simulink model "NORTest"  (R2016a)
settings: Solver=VariableStepAuto  StartTime=0.0  StopTime=1  RelTol=1e-3
libraries: SimscapeMacros x5, elec_lib x2, fl_lib x1, ProjectBlocks x1, nesl_utility x1
settings Model: Creator=Peter  LastModifiedBy=Peter

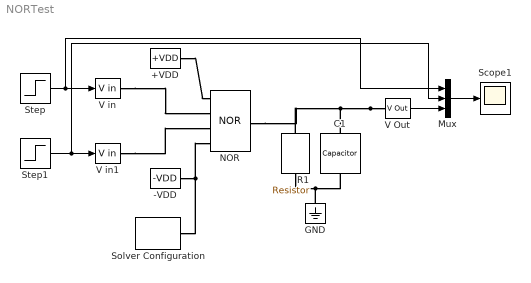
== system NORTest ==
  +VDD : SimscapeMacros/+VDD
  -VDD : SimscapeMacros/-VDD
  C1 : elec_lib/Passive Devices/Capacitor  enable_table=0  c=1e-6 F  Cvec=[ 1e-5 1e-6 ] F  Vvec=[ 0 10 ] V  CV_table_symmetry=1  C_tol=5  enable_C_tol=0  tol_distribution=1  nSigma=4  r=1e-6 Ohm  g=0 1/Ohm  initV=0 V  enable_operating_limits=0  operating_limit_action=1  max_working_voltage_range=[ -25 25 ] V  power_rating=1 W  enable_faults=0  fault_action=1  Cscale_faulted=100  R_faulted=0.001 Ohm  G_faulted=0 1/Ohm  tau_fault=0.001 s  enable_temporal_fault=0  t_fault=1 s  enable_behavioral_fault=0  max_permissible_voltage_range=[ -100 100 ] V  t_fail_on_voltage=1 s
  GND : fl_lib/Electrical/Electrical Elements/Electrical Reference
  Mux : Mux  Inputs=3
  NOR : ProjectBlocks/NOR
  R1 : elec_lib/Passive Devices/Resistor  R=10e3 Ohm  R_tol=5  enable_R_tol=0  tol_distribution=1  nSigma=4  enable_operating_limits=0  operating_limit_action=2  max_working_voltage=100 V  power_rating=1 W  enable_faults=0  fault_action=1  R_faulted=Inf Ohm  enable_temporal_fault=0  t_fault=1 s  enable_behavioral_fault=0  max_permissible_current=1 A  t_fail_on_current=1 s  noise_mode=0  sample_time=0.001 s  repeatability=1  auto_seed=359705264  user_seed=0  Tdevice=25 degC  alpha=0.00393 1/K  Tmeas=25 degC  thermal_mass=100 J/K  initial_temperature=25 degC  power_derating_T1=70 degC  power_derating_T2=155 degC  operating_temperature_range_vec=[ -50 150 ] degC
  Scope1 : Scope
  Solver Configuration : nesl_utility/Solver Configuration  PhysicalDomain=network_engine_domain  SubClassName=solver  LeftPortType=input  RightPortType=generic  Accelerate=off  Tones=[]  Harmonics=[]  SimulateNoise=off  Profile=off  UseLocalSampling=off  EnableSwitchedLinearOptims=on  FrequencyDomain=off  UseCCode=off  RelTol=0.001  AbsTol=1e-06  MinStep=1e-09  ToWorkspace=off  RevertToSquareIcSolve=off  NumHomotopyIterations=100  PhasorMode=off  PhasorModeNumHarmonics=1  OverrideAbsTol=off  DoDC=off  ResidualTolerance=1e-09  UseLocalSolver=off  LocalSolverChoice=NE_BACKWARD_EULER_ADVANCER  LocalSolverSampleTime=0.001  DoFixedCost=off  MaxNonlinIter=3  MaxModeIter=2  LinearAlgebra=Sparse  DelaysMemoryBudget=1024  AutomaticFiltering=on  FilteringTimeConstant=0.001
  Step : Step  Time=.5  Before=-10  After=10  SampleTime=0
  Step1 : Step  Time=.25  Before=10  After=-10  SampleTime=0
  V Out : SimscapeMacros/V Out
  V in : SimscapeMacros/V in
  V in1 : SimscapeMacros/V in
  wires:
  Step/1 -> V in/1, Mux/1
  Mux/1 -> Scope1/1
  Step1/1 -> Mux/2, V in1/1
  V Out/1 -> Mux/3
  connections:
  V Out/LConn1 -- NOR/RConn1 -- R1/LConn1 -- C1/LConn1
  GND/LConn1 -- R1/RConn1 -- C1/RConn1
  V in/RConn1 -- NOR/LConn2
  V in1/RConn1 -- NOR/LConn3
  +VDD/RConn1 -- NOR/LConn1
  -VDD/RConn1 -- NOR/LConn4 -- Solver Configuration/RConn1
